simulink model "fuzzy_control_t1"  (R2017a)
settings: Solver=VariableStepAuto  StartTime=0.0  StopTime=10.0  FixedStep=0.001  RelTol=1e-3
undefined symbols (not defined in the file or in its folder): DiscIntNeverNeededParam
libraries: simulink x4, fuzblock x1
settings Model: Creator=Chaohua Zhao  LastModifiedBy=Chaohua Zhao

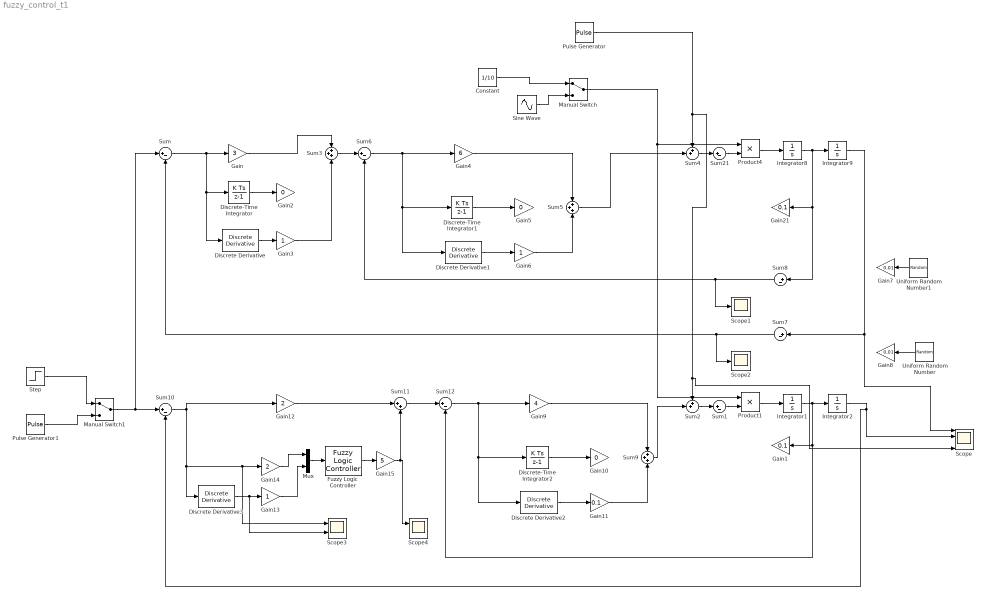
== system fuzzy_control_t1 ==
  Constant : Constant  Value=1/10
  Discrete Derivative : simulink/Discrete/Discrete Derivative  gainval=1.0  ICPrevScaledInput=0.0  OutMin=[]  OutMax=[]  OutDataType=fixdt(1, 16)  OutScaling=2^-10  DoSatur=off
  Discrete Derivative1 : simulink/Discrete/Discrete Derivative  gainval=1.0  ICPrevScaledInput=0.0  InputProcessing=Inherited  OutMin=[]  OutMax=[]  OutDataType=fixdt(1, 16)  OutScaling=2^-10  DoSatur=off
  Discrete Derivative2 : simulink/Discrete/Discrete Derivative  gainval=1.0  ICPrevScaledInput=0.0  InputProcessing=Inherited  OutMin=[]  OutMax=[]  OutDataType=fixdt(1, 16)  OutScaling=2^-10  DoSatur=off
  Discrete Derivative3 : simulink/Discrete/Discrete Derivative  gainval=1.0  ICPrevScaledInput=0.0  InputProcessing=Inherited  OutMin=[]  OutMax=[]  OutDataType=fixdt(1, 16)  OutScaling=2^-10  DoSatur=off
  Discrete-Time Integrator : DiscreteIntegrator  InitialConditionSetting=State (most efficient)  SampleTime=-1  ICPrevOutput=DiscIntNeverNeededParam  ICPrevScaledInput=DiscIntNeverNeededParam
  Discrete-Time Integrator1 : DiscreteIntegrator  InitialConditionSetting=State (most efficient)  SampleTime=-1  ICPrevOutput=DiscIntNeverNeededParam  ICPrevScaledInput=DiscIntNeverNeededParam
  Discrete-Time Integrator2 : DiscreteIntegrator  InitialConditionSetting=State (most efficient)  SampleTime=-1  ICPrevOutput=DiscIntNeverNeededParam  ICPrevScaledInput=DiscIntNeverNeededParam
  Fuzzy Logic Controller : fuzblock/Fuzzy Logic  Controller  fis=['fuzzy_sug_t2']
  Gain : Gain  Gain=3
  Gain1 : Gain  Gain=0.1
  Gain10 : Gain  Gain=0
  Gain11 : Gain  Gain=0.1
  Gain12 : Gain  Gain=2
  Gain13 : Gain
  Gain14 : Gain  Gain=2
  Gain15 : Gain  Gain=5
  Gain2 : Gain  Gain=0
  Gain21 : Gain  Gain=0.1
  Gain3 : Gain
  Gain4 : Gain  Gain=6
  Gain5 : Gain  Gain=0
  Gain6 : Gain
  Gain7 : Gain  Gain=0.01
  Gain8 : Gain  Gain=0.01
  Gain9 : Gain  Gain=4
  Integrator{1..2,8..9} (4 alike) : Integrator
  Manual Switch : ManualSwitch
  Manual Switch1 : ManualSwitch
  Mux : Mux  Inputs=2
  Product1 : Product
  Product4 : Product
  Pulse Generator : DiscretePulseGenerator  PulseType=Time based  Period=3  PulseWidth=4  PhaseDelay=5
  Pulse Generator1 : DiscretePulseGenerator  PulseType=Time based  Period=15  PulseWidth=50
  Scope : Scope  NumInputPorts=4
  Scope1 : Scope
  Scope2 : Scope
  Scope3 : Scope  NumInputPorts=2
  Scope4 : Scope  NumInputPorts=2
  Sine Wave : Sin  Amplitude=0.4  Bias=0.5  SampleTime=0
  Step : Step  Time=0  After=3  SampleTime=0
  Sum{,1,6..8,10,12,21} (8 alike) : Sum  Inputs=|+-
  Sum11 : Sum  Inputs=|++
  Sum2 : Sum  Inputs=++|
  Sum3 : Sum  Inputs=+++
  Sum4 : Sum  Inputs=++|
  Sum5 : Sum  Inputs=+++
  Sum9 : Sum  Inputs=+++
  Uniform Random Number : UniformRandomNumber  SampleTime=0.001
  Uniform Random Number1 : UniformRandomNumber  SampleTime=0.001
  wires:
  Integrator8/1 -> Integrator9/1, Sum8/1, Gain21/1
  Sum4/1 -> Sum21/1
  Sum21/1 -> Product4/2
  Product4/1 -> Integrator8/1
  Sine Wave/1 -> Manual Switch/2
  Constant/1 -> Manual Switch/1
  Product1/1 -> Integrator1/1
  Sum1/1 -> Product1/2
  Sum2/1 -> Sum1/1
  Integrator1/1 -> Integrator2/1, Gain1/1, Sum12/2
  Step/1 -> Manual Switch1/1
  Pulse Generator1/1 -> Manual Switch1/2
  Integrator9/1 -> Sum7/1, Scope/1
  Gain4/1 -> Sum5/1
  Discrete Derivative1/1 -> Gain6/1
  Discrete-Time Integrator1/1 -> Gain5/1
  Sum6/1 -> Gain4/1, Discrete Derivative1/1, Discrete-Time Integrator1/1
  Sum5/1 -> Sum4/2
  Sum3/1 -> Sum6/1
  Discrete Derivative/1 -> Gain3/1
  Discrete-Time Integrator/1 -> Gain2/1
  Gain/1 -> Sum3/1
  Sum/1 -> Discrete Derivative/1, Discrete-Time Integrator/1, Gain/1
  Gain3/1 -> Sum3/3
  Uniform Random Number/1 -> Gain8/1
  Uniform Random Number1/1 -> Gain7/1
  Sum8/1 -> Scope1/1, Sum6/2
  Sum7/1 -> Scope2/1, Sum/2
  Sum9/1 -> Sum2/2
  Mux/1 -> Fuzzy Logic Controller/1
  Gain13/1 -> Mux/2
  Gain14/1 -> Mux/1
  Sum10/1 -> Discrete Derivative3/1, Scope3/1, Gain14/1, Gain12/1
  Fuzzy Logic Controller/1 -> Gain15/1
  Integrator2/1 -> Sum10/2, Scope/2
  Gain15/1 -> Sum11/2, Scope4/1
  Discrete Derivative3/1 -> Scope3/2, Gain13/1
  Gain6/1 -> Sum5/3
  Gain11/1 -> Sum9/3
  Sum12/1 -> Discrete-Time Integrator2/1, Discrete Derivative2/1, Gain9/1
  Discrete-Time Integrator2/1 -> Gain10/1
  Discrete Derivative2/1 -> Gain11/1
  Gain9/1 -> Sum9/1
  Manual Switch1/1 -> Sum/1, Sum10/1
  Manual Switch/1 -> Product4/1, Product1/1
  Pulse Generator/1 -> Scope/4, Sum2/1, Sum4/1
  Gain12/1 -> Sum11/1
  Sum11/1 -> Sum12/1
